simulink model "sensorsAndActuators"  (R2024a)
settings: Solver=ode2  StartTime=0.0  StopTime=inf  FixedStep=1/500  RelTol=1e-3  EnableMultiTasking=on
undefined symbols (not defined in the file): gcbh, HIL, JPEG, qc_get_step_size, video_display_show
libraries: quarc_library x32, simulink x4, simulink_extras x1
settings Model: ExtModeTrigDuration=10000  Creator=Lorena Gonzalez  LastModifiedBy=Lorena Gonzalez
settings SolverCC: AlgebraicLoopSolver=TrustRegion  PositivePriorityOrder=on
settings DataIOCC: ReturnWorkspaceOutputs=off
settings DebuggingCC: UnconnectedInputMsg=warning  UnconnectedOutputMsg=warning  UnconnectedLineMsg=warning  ArithmeticOperatorsInVariantConditions=warning
settings ModelReferenceCC: EnableRefExpFcnMdlSchedulingChecks=on
settings SFSimCC: SimUseLocalCustomCode=off  CustomCodeUndefinedFunction=UseInterfaceOnly
settings RTWCC: Description=QUARC Win64 Target Using Toolchain  SystemTargetFile=quarc_win64.tlc  TemplateMakefile=quarc_default_tmf  RTWUseLocalCustomCode=off  Toolchain=QUARC win64 | nmake (64-bit Windows)  BuildConfiguration=Faster Runs  GPUComputeCapability=3.5
settings CodeAppCC: StateflowObjectComments=on
settings STFCustomTargetCC: ConcurrentExecutionCompliant=on  SystemTargetFile=quarc_win64.tlc
settings GRTTargetCC: ParMdlRefBuildCompliant=off  CompOptLevelCompliant=off  CombineOutputUpdateFcns=off  MatFileLogging=off  CPPClassGenCompliant=off  GRTInterface=on  ExtMode=on  ExtModeMexFile=quarc_comm
settings ConfigComp: CovMetricSettings=dswe

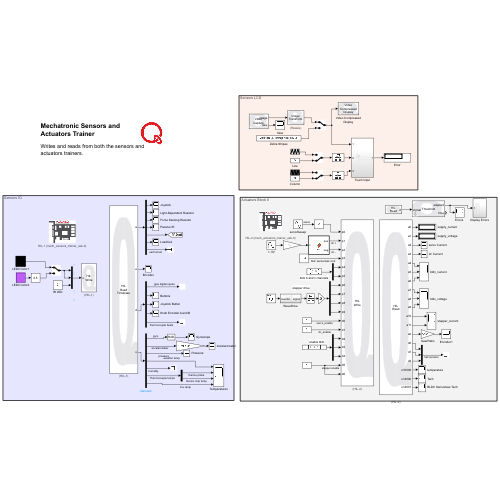
[thumbnail: Simulink's stored preview of the top-level diagram]
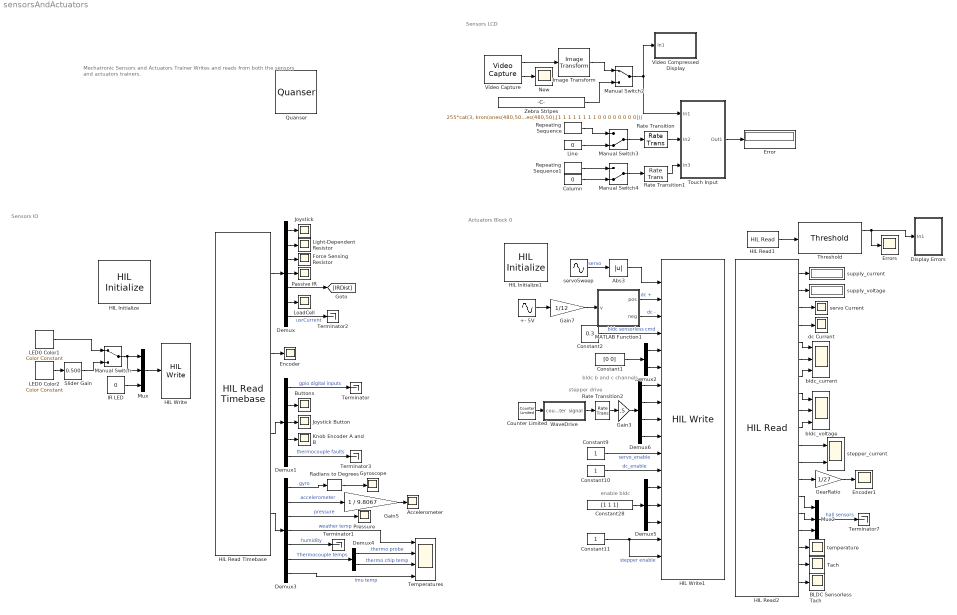
== system sensorsAndActuators ==
  note: Sensors IO
  note: Mechatronic Sensors and Actuators Trainer
      |
      | Writes and reads from both the sensors and actuators trainers.
  note: Sensors LCD
  note: enable bldc
  note: bldc b and c channels
  note: stepper drive
  note: Actuators Block 0
  +- 5V : Sin  Amplitude=5  Frequency=.75  SampleTime=0
  Abs3 : Abs  SaturateOnIntegerOverflow=off
  Accelerometer : Scope
  BLDC Sensorless Tach : Scope
  Buttons : Scope
  Column : Constant  Value=0
  Constant1 : Constant  Value=[0 0]
  Constant10 : Constant
  Constant11 : Constant
  Constant2 : Constant  Value=0.3
  Constant28 : Constant  Value=[1 1 1]
  Constant9 : Constant
  Counter Limited : simulink/Sources/Counter Limited  uplimit=3  tsamp=1/100
  Demux : Demux  Outputs=[2 1 1 1 1 1 1]
  Demux1 : Demux  Outputs=[4 2 1 2 4]
  Demux2 : Demux  Outputs=2
  Demux3 : Demux  Outputs=[3 3 1 1 2 1 1]
  Demux4 : Demux  Outputs=2
  Demux5 : Demux  Outputs=3
  Demux6 : Demux
  Display Errors : Subsystem
  Encoder : Scope
  Encoder1 : Scope
  Error : Display
  "Errors " : Scope
  Force Sensing Resistor : Scope
  Gain3 : Gain  Gain=.5
  Gain5 : Gain  Gain=1 / 9.8067
  Gain7 : Gain  Gain=1/12
  GearRatio : Gain  Gain=1/27
  Gyroscope : Scope
  HIL Initialize : quarc_library/Data Acquisition/Generic/Configuration/HIL Initialize  object_name=HIL-1  board_type=mech_sensors_trainer_usb  board_number=0  board_options=accel_avg=1;accel_filter=246;accel_fs=16;accel_rate=1125;adc1_os=64;adc2_os=64;adc3_os=16;btn0_pol=1;btn1_pol=1;color_ag=4.0;color_dg=4;color_int=50;dio0_mode=digital;dio1_mode=digital;dio2_mode=digital;dio3_mode=digital;enc_dir=0;enc_mode=encoder;enc_freq=240000000;gyro_avg=1;gyro_filter=196.6;gyro_fs=2000;gyro_rate=1125;hum_over=2;knob_dir=0;load_gain=128;load_rate=320;press_over=4;radar_bins=0;radar_down=1;radar_gain=0.3;radar_hwaas=30;radar_len=1;radar_mur=6;radar_noise=0;radar_prof=3;radar_run=0.7;radar_samp=A;radar_serv=none;radar_start=0.2;radar_sweeps=16;radar_swprate=0;temp_filter=7932;temp_over=8;tof_freq=15;tof_int=2;tof_order=close;tof_res=8x8;tof_sharp=14;ultra_int=100;ultra_len=2.4;ultra_serv=none;ultra_start=0;weather_filt=2;weather_standby=0.5;  exclusive=off  active=on  hardware_clocks=[0]  clock_modes=[]  initial_clock_frequencies=[]  set_clock_params_at_start=off  set_clock_params_at_switch_in=off  set_clock_frequencies_at_start=off  set_clock_frequencies_at_switch_in=off  analog_input_channels=[0:11]  analog_input_configurations=[]  analog_input_maximums=3.3  analog_input_minimums=0  set_analog_input_params_at_start=off  set_analog_input_params_at_switch_in=off  analog_output_channels=[]  analog_output_maximums=[]  analog_output_minimums=[]  initial_analog_outputs=[]  final_analog_outputs=[]  watchdog_analog_outputs=[]  set_analog_output_params_at_start=off  set_analog_output_params_at_switch_in=off  set_analog_outputs_at_start=off  set_analog_outputs_at_switch_in=off  set_analog_outputs_at_terminate=off  set_analog_outputs_at_switch_out=off  set_analog_outputs_on_watchdog=off  digital_input_channels=[0:30]  digital_output_channels=[]  digital_output_configuration=[]  initial_digital_outputs=[0]  final_digital_outputs=[0]  watchdog_digital_outputs=[0]  set_digital_output_params_at_start=off  set_digital_output_params_at_switch_in=off  set_digital_outputs_at_start=on  set_digital_outputs_at_switch_in=off  set_digital_outputs_at_terminate=on  set_digital_outputs_at_switch_out=off  set_digital_outputs_on_watchdog=on  encoder_channels=[0:1]  quadrature=[4]  encoder_filter_frequency=[240e6]  initial_encoder_counts=[0]  set_encoder_params_at_start=on  set_encoder_params_at_switch_in=off  set_encoder_counts_at_start=on  set_encoder_counts_at_switch_in=off  pwm_channels=[]  pwm_modes=[0]  pwm_frequency=14648.4375  pwm_configuration=[0]  pwm_alignment=[0]  pwm_polarity=[1]  pwm_leading_deadband=[]  pwm_trailing_deadband=[]  initial_pwm_outputs=[0]  final_pwm_outputs=[0]  watchdog_pwm_outputs=[0]  set_pwm_params_at_start=on  set_pwm_params_at_switch_in=off  set_pwm_outputs_at_start=on  set_pwm_outputs_at_switch_in=off  set_pwm_outputs_at_terminate=on  set_pwm_outputs_at_switch_out=off  set_pwm_outputs_on_watchdog=on  other_output_channels=[11000:11012]  initial_other_outputs=[0]  final_other_outputs=[0]  watchdog_other_outputs=[0]  set_other_outputs_at_start=on  set_other_outputs_at_switch_in=off  set_other_outputs_at_terminate=on  set_other_outputs_at_switch_out=off  set_other_outputs_on_watchdog=on
  HIL Initialize1 : quarc_library/Data Acquisition/Generic/Configuration/HIL Initialize  object_name=HIL-2  board_type=mech_actuators_trainer_usb  board_number=0  board_options=supply_voltage_low_limit=10.0;supply_voltage_high_limit=16.0;supply_current_high_limit=8.0;dc_motor_current_high_limit=1.1;servo_motor_current_high_limit=1.3;bldc_motor_current_high_limit=2.0;stepper_motor_current_high_limit=1.7;servo_pwm_range=0;enc_dir=0;bldc_motor_mode=1;bldc_start_tc=0.03;bldc_start_target=1200  exclusive=off  active=on  hardware_clocks=[0]  clock_modes=[]  initial_clock_frequencies=[]  set_clock_params_at_start=off  set_clock_params_at_switch_in=off  set_clock_frequencies_at_start=off  set_clock_frequencies_at_switch_in=off  analog_input_channels=[0:11]  analog_input_configurations=[]  analog_input_maximums=3  analog_input_minimums=-3  set_analog_input_params_at_start=off  set_analog_input_params_at_switch_in=off  analog_output_channels=[]  analog_output_maximums=[]  analog_output_minimums=[]  initial_analog_outputs=[]  final_analog_outputs=[]  watchdog_analog_outputs=[]  set_analog_output_params_at_start=off  set_analog_output_params_at_switch_in=off  set_analog_outputs_at_start=off  set_analog_outputs_at_switch_in=off  set_analog_outputs_at_terminate=off  set_analog_outputs_at_switch_out=off  set_analog_outputs_on_watchdog=off  digital_input_channels=[0:17]  digital_output_channels=[0:6]  digital_output_configuration=[]  initial_digital_outputs=[1]  final_digital_outputs=[0]  watchdog_digital_outputs=[0]  set_digital_output_params_at_start=off  set_digital_output_params_at_switch_in=off  set_digital_outputs_at_start=on  set_digital_outputs_at_switch_in=off  set_digital_outputs_at_terminate=on  set_digital_outputs_at_switch_out=off  set_digital_outputs_on_watchdog=on  encoder_channels=[0]  quadrature=[4]  encoder_filter_frequency=[]  initial_encoder_counts=[0]  set_encoder_params_at_start=on  set_encoder_params_at_switch_in=off  set_encoder_counts_at_start=on  set_encoder_counts_at_switch_in=off  pwm_channels=[0:9]  pwm_modes=[0]  pwm_frequency=23195  pwm_configuration=[1]  pwm_alignment=[0]  pwm_polarity=[1]  pwm_leading_deadband=[0]  pwm_trailing_deadband=[0]  initial_pwm_outputs=[0]  final_pwm_outputs=[0]  watchdog_pwm_outputs=[0]  set_pwm_params_at_start=off  set_pwm_params_at_switch_in=off  set_pwm_outputs_at_start=on  set_pwm_outputs_at_switch_in=off  set_pwm_outputs_at_terminate=on  set_pwm_outputs_at_switch_out=off  set_pwm_outputs_on_watchdog=on  other_output_channels=[]  initial_other_outputs=[]  final_other_outputs=[]  watchdog_other_outputs=[]  set_other_outputs_at_start=off  set_other_outputs_at_switch_in=off  set_other_outputs_at_terminate=off  set_other_outputs_at_switch_out=off  set_other_outputs_on_watchdog=off
  HIL Read Timebase : quarc_library/Data Acquisition/Generic/Timebases/HIL Read Timebase  object_name=HIL-1  clock=0  analog_channels=0:7  encoder_channels=0:1  digital_channels=[0:12]  other_channels=[3000:3002 4000:4002 9000 10000:10003 11000]  active=on  vector_output=on  data_type_mode=Inherit via back propagation  encoder_data_type=double  digital_data_type=boolean  overflow_mode=Error on overflow  samples_in_buffer=max(ceil(1/qc_get_step_size), 1)
  HIL Read1 : quarc_library/Data Acquisition/Generic/Immediate I//O/HIL Read  object_name=HIL-2  analog_channels=[]  encoder_channels=[]  digital_channels=[3:17]  other_channels=[]  sample_time=qc_get_step_size  active=on  vector_output=on  data_type_mode=Inherit via back propagation  encoder_data_type=double  digital_data_type=boolean
  HIL Read2 : quarc_library/Data Acquisition/Generic/Immediate I//O/HIL Read  object_name=HIL-2  analog_channels=[0:11]  encoder_channels=[0]  digital_channels=[0:2]  other_channels=[10000 14000:14001]  sample_time=qc_get_step_size  active=on  vector_output=off  data_type_mode=Inherit via back propagation  encoder_data_type=double  digital_data_type=boolean
  HIL Write : quarc_library/Data Acquisition/Generic/Immediate I//O/HIL Write  object_name=HIL-1  analog_channels=[]  pwm_channels=[]  digital_channels=[]  other_channels=[11000:11006]  sample_time=-1  active=off  vector_input=on
  HIL Write1 : quarc_library/Data Acquisition/Generic/Immediate I//O/HIL Write  object_name=HIL-2  analog_channels=[]  pwm_channels=[0:9]  digital_channels=[0:6]  other_channels=[]  sample_time=-1  active=off  vector_input=off
  IR LED : Constant  Value=0
  Image Transform : quarc_library/Image Processing/Generic/Image Transform  algorithm=Resize  color_theme=KRYGCBMW  min_pixel=0  max_pixel=4000  contour_depth=1  focal_length=308  principal_point=[262 334]  radial_coeffs=[-0.3129 0.0907]  tangential_coeffs=[]  extrapolated_pixel=0  interpolation=nearest  row_coords=0  column_coords=0  output_height=480  output_width=800  angle=0  origin=[240 320]  output_origin=[240 320]  output_data_type=uint8
      settings: AttributesFormatString=(%<algorithm>)  SourceProductName=QUARC Targets
  Joystick : Scope
  Joystick Button : Scope
  Knob Encoder A and B : Scope
  LED0 Color1 : quarc_library/Sources/Signals/Color Constant  color=[1 0.8 1]*0
      settings: SourceProductName=QUARC Targets
  LED0 Color2 : quarc_library/Sources/Signals/Color Constant  color=[0.75 0.36 0.98]
      settings: SourceProductName=QUARC Targets
  Light-Dependent Resistor : Scope
  Line : Constant  Value=0
  LoadCell : Scope
  MATLAB Function1 : MATLAB Function  TreatAsAtomicUnit=on
  Manual Switch : ManualSwitch
  Manual Switch2 : ManualSwitch
  Manual Switch3 : ManualSwitch  CurrentSetting=0
  Manual Switch4 : ManualSwitch  CurrentSetting=0
  Mux : Mux  Inputs=[3,3,1]
  Mux2 : Mux  Inputs=3
  New : Scope
  Passive IR : Scope
  Pressure : Scope
  Quanser : quarc_library/Logos/Quanser
  Radians to Degrees : simulink_extras/Transformations/Radians to Degrees
  Rate Transition : RateTransition  OutPortSampleTime=qc_get_step_size * ceil(1 / 30 / qc_get_step_size)
  Rate Transition1 : RateTransition  OutPortSampleTime=qc_get_step_size * ceil(1 / 30 / qc_get_step_size)
  Rate Transition2 : RateTransition
  Repeating Sequence : simulink/Sources/Repeating Sequence  rep_seq_t=[0 5 10]/5  rep_seq_y=[-200 200 -200]
  Repeating Sequence1 : simulink/Sources/Repeating Sequence  rep_seq_t=([0 5 10 15 20])/7  rep_seq_y=[-120 120 -120 120 -120]
  Slider Gain : simulink/Math Operations/Slider Gain  gain=0.500  low=0  high=1
  Tach : Scope
  Temperatures : Scope  NumInputPorts=4
  Terminator{,1..3,7} (5 alike) : Terminator
  Threshold : quarc_library/Discontinuities/Threshold  operator=>  param_src=Specify via dialog  threshold=0  duration=0.02
      settings: SourceProductName=QUARC Targets
  Touch Input : Subsystem
  Video Capture : quarc_library/Multimedia/Video Capture  source=device  device=0  filename=sample_movie.mov  value=[0 0; 0 0]  resolution=640 x 480  width=640  height=480  output_format=MATLAB RGB (HxWx3)  data_type=uint8  sample_time=qc_get_step_size * ceil(1 / 30.0 / qc_get_step_size)  brightness_override=Do not override  brightness=50.0  contrast_override=Do not override  contrast=50.0  hue_override=Do not override  hue=50.0  saturation_override=Do not override  saturation=50.0  sharpness_override=Do not override  sharpness=50.0  gamma_override=Do not override  gamma=50.0  coloreffect_override=Do not override  coloreffect=None  whitebalance_override=Do not override  whitebalance=50.0  backlightcompensation_override=Do not override  backlightcompensation=0.0  gain_override=Do not override  gain=50.0  pan_override=Do not override  pan=50.0  tilt_override=Do not override  tilt=50.0  roll_override=Do not override  roll=50.0  zoom_override=Do not override  zoom=0.0  exposure_override=Do not override  exposure=50.0  iris_override=Do not override  iris=50.0  mirror_override=Do not override  mirror=None  focus_override=Do not override  focus=0.0
      settings: SourceProductName=QUARC Targets
  Video Compressed Display : Subsystem  LoadFcn=set_param(gcbh, 'UserData', gcb);  StartFcn=video_display_show([gcb, '/Video Display'], 'add', gcb);  mask(Video Compressed Display){algorithm=JPEG, quality=50, sample_time=-1, use_hardware=on}
      mask prompts: algorithm "Compression algorithm:"; quality "Compression quality (0-100):"; sample_time "Sample time (seconds):"; use_hardware "Use hardware acceleration for video display"
      mask help: Displays a video stream on the host, using compression to minimize bandwidth.
      mask init:
      | qc_set_display('Video\nCompressed\nDisplay');
      settings: UndoDeleteFcn=set_param(gcbh, 'UserData', gcb);  OpenFcn=video_display_show([gcb, '/Video Display'], 'show', gcb);  PreDeleteFcn=video_display_show([gcb, '/Video Display'], 'delete');
      settings: CopyFcn=|
      | set_param(gcbh, 'UserData', gcb);
      | set_param(gcbh, 'LinkStatus', 'none');
      settings: NameChangeFcn=|
      | video_display_show([get_param(gcbh, 'UserData'), '/Video Display'], 'rename', [gcb, '/Video Display']);
      | video_display_show([gcb, '/Video Display'], 'add', gcb);
      | set_param(gcbh, 'UserData', gcb);
      mask Help: web(qc_get_block_help_path(gcb));
      mask TypeOptions algorithm: Image Compress/algorithm
      mask TypeOptions quality: Image Compress/quality
      mask TypeOptions sample_time: Video Display/sample_time
      mask TypeOptions use_hardware: Video Display/use_hardware
      mask Display:
      | patch([0.98591 0.98591 0.62618 0.59072 0.56147   0.536   0.536  0.5441 0.56912 0.59207 0.60881 0.62276 0.63527 0.64364  0.6485  0.6485 0.64706 0.64499 0.63662 0.62411 0.61232 0.59837 0.58307 0.56147   0.536   0.536  0.5441  0.5747 0.60953 0.63662 0.67001  0.7034 0.72851 0.75425 0.77927 0.80294 0.82454 0.84119 0.85865 0.87395 0.88574 0.89339  0.8969 0.89969 0.89969 0.89267  0.8816 0.87044 0.85649  0.8384 0.81824 0.80294 0.78764 0.77513 0.76676 0.75776 0.76397 0.77513 0.79178 0.80987 0.82796 0.84326 0.86207 0.98528],[0.18689 0.05522 0.05522 0.05171 0.05171    0.05 0.18338 0.18338 0.19148 0.20435 0.22298 0.24863 0.28589 0.33125 0.38138 0.55139 0.59801 0.63761 0.68189 0.72149 0.74939 0.76694 0.77855 0.79367 0.79952 0.92768 0.92768 0.92768 0.92417 0.92066 0.91364  0.9032 0.89384 0.88106 0.86594 0.85073 0.82634 0.80537 0.77855 0.74363 0.70403 0.65858 0.61079 0.59099 0.41513 0.37202 0.31847 0.29048 0.25556 0.23342  0.2102 0.19382 0.18221 0.17285 0.16943 0.16124  0.1589 0.16241 0.16709 0.17168  0.1787 0.18221 0.18689 0.18689],[0.9,0.90,0.91])
      | patch([0.536 0.52601 0.46823 0.44528 0.41603 0.39101 0.35555 0.33116 0.31451 0.29291  0.2804 0.26717 0.25322 0.23999 0.22406 0.20732 0.19337 0.17528 0.15935 0.14396 0.13217 0.11759 0.10922 0.10085 0.09671 0.09392 0.09041 0.08906 0.08906 0.09464  0.0995 0.10778 0.11894 0.13145 0.14675 0.16349 0.17672 0.19409 0.20732 0.22406 0.23999 0.26159 0.27833 0.29849 0.31793 0.33602 0.35411 0.37085 0.39245 0.41603   0.536   0.536 0.53159 0.46409   0.446 0.42026 0.39587 0.37571 0.36113 0.34925 0.34088 0.33809 0.33809 0.34088 0.34583 0.35627 0.36392 0.38129 0.39587 0.41117 0.42719 0.44672  0.4676 0.48353 0.48353 0.52394   0.536],[0.05 0.04829 0.04712 0.04712 0.04829 0.05063 0.05405 0.05873 0.06107 0.06692 0.07043 0.07619 0.08087 0.08672 0.09482 0.10652 0.11696 0.13325  0.1508 0.17168 0.19499 0.22415 0.25439 0.28472 0.31379 0.35456 0.38489 0.41513 0.58055 0.63878 0.68774 0.72149 0.75641 0.78089 0.80537 0.82859 0.84029 0.85658 0.86594 0.87404  0.8834 0.89267 0.90086 0.90788 0.91247 0.91832 0.92066   0.923 0.92651 0.92768 0.92768 0.79952 0.79952 0.79952 0.79718 0.78899 0.77153 0.75056 0.72149 0.68072 0.62249  0.5549 0.41396 0.37085 0.33242 0.28121 0.25205 0.22181 0.20552 0.19499 0.18572 0.18221 0.17753 0.17636 0.17753  0.1787  0.1787],[0.9,0.90,0.91])
      | disp('Video\nCompressed\nDisplay');
  WaveDrive : Subsystem
  Zebra Stripes : Constant  Value=255*cat(3, kron(ones(480,50),[1 1 1 1 1 1 1 1 0 0 0 0 0 0 0 0]),kron(ones(480,50),[1 1 1 1 1 1 1 1 0 0 0 0 0 0 0 0]),kron(ones(480,50),[1 1 1 1 1 1 1 1 0 0 0 0 0 0 0 0]))  OutDataTypeStr=uint8
  bldc_current : Scope  NumInputPorts=3
  bldc_voltage : Scope  NumInputPorts=3
  dc Current : Scope
  servo Current : Scope
  servoSweep : Sin  SampleTime=0
  stepper_current : Scope  NumInputPorts=2
  supply_current : Display
  supply_voltage : Display
  temperature : Scope
  wires:
  Rate Transition1/1 -> Touch Input/3(In3)
  Video Capture/1 -> Image Transform/1
  Demux3/2 -> Gain5/1  "accelerometer"
  Image Transform/1 -> Manual Switch2/1
  Radians to Degrees/1 -> Gyroscope/1
  Manual Switch3/1 -> Rate Transition/1
  Demux/7 -> Terminator2/1  "usrCurrent"
  Demux1/5 -> Terminator3/1  "thermocouple faults"
  Repeating Sequence1/1 -> Manual Switch4/1
  Repeating Sequence/1 -> Manual Switch3/1
  Demux4/1 -> Temperatures/2  "thermo probe"
  Demux1/4 -> Knob Encoder A and B/1
  Touch Input/1(Out1) -> Error/1
  Rate Transition/1 -> Touch Input/2(In2)
  HIL Read Timebase/1 -> Demux/1
  Slider Gain/1 -> Manual Switch/2
  Demux/6 -> LoadCell/1
  Demux1/1 -> Terminator/1  "gpio digital inputs"
  Demux/3 -> Force Sensing Resistor/1
  Demux3/1 -> Radians to Degrees/1  "gyro"
  LED0 Color2/1 -> Slider Gain/1
  LED0 Color1/1 -> Manual Switch/1
  Manual Switch/1 -> Mux/2, Mux/1
  Demux/2 -> Light-Dependent Resistor/1
  Demux3/6 -> Demux4/1  "Thermocouple temps"
  Demux4/2 -> Temperatures/3  "thermo chip temp"
  IR LED/1 -> Mux/3
  Gain5/1 -> Accelerometer/1
  Demux1/3 -> Joystick Button/1
  Video Capture/2 -> New/1
  Demux/5 -> [IRDist]
  Demux/1 -> Joystick/1
  Line/1 -> Manual Switch3/2
  Manual Switch4/1 -> Rate Transition1/1
  Demux3/3 -> Pressure/1  "pressure"
  Mux/1 -> HIL Write/1
  Demux/4 -> Passive IR/1
  Demux3/4 -> Temperatures/1  "weather temp"
  Demux3/7 -> Temperatures/4  "imu temp"
  HIL Read Timebase/2 -> Encoder/1
  Manual Switch2/1 -> Touch Input/1(In1), Video Compressed Display/1(In1)
  HIL Read Timebase/3 -> Demux1/1
  Zebra Stripes/1 -> Manual Switch2/2
  Column/1 -> Manual Switch4/2
  HIL Read Timebase/4 -> Demux3/1
  Demux1/2 -> Buttons/1
  HIL Read2/18 -> Tach/1
  Abs3/1 -> HIL Write1/1
  HIL Read2/4 -> dc Current/1
  HIL Read2/19 -> BLDC Sensorless Tach/1
  Demux5/1 -> HIL Write1/13
  Demux5/2 -> HIL Write1/14
  Threshold/1 -> Display Errors/1(In1), "Errors "/1
  GearRatio/1 -> Encoder1/1
  Constant11/1 -> HIL Write1/16, HIL Write1/17  "stepper enable"
  Constant9/1 -> HIL Write1/11  "servo_enable"
  MATLAB Function1/2(neg) -> HIL Write1/3  "dc -"
  MATLAB Function1/1(pos) -> HIL Write1/2  "dc +"
  Demux6/2 -> HIL Write1/8
  Demux2/2 -> HIL Write1/6
  HIL Read2/12 -> stepper_current/2
  Demux2/1 -> HIL Write1/5
  HIL Read2/13 -> GearRatio/1
  Gain7/1 -> MATLAB Function1/1(v)
  Gain3/1 -> Demux6/1
  servoSweep/1 -> Abs3/1  "servo"
  +- 5V/1 -> Gain7/1
  WaveDrive/1(signal) -> Rate Transition2/1
  Demux6/3 -> HIL Write1/9
  Mux2/1 -> Terminator7/1  "hall sensors"
  HIL Read2/10 -> bldc_voltage/3
  HIL Read2/17 -> temperature/1
  HIL Read2/8 -> bldc_voltage/1
  HIL Read2/9 -> bldc_voltage/2
  Constant28/1 -> Demux5/1
  Demux5/3 -> HIL Write1/15
  HIL Read2/16 -> Mux2/3
  Counter Limited/1 -> WaveDrive/1(counter)
  Constant2/1 -> HIL Write1/4  "bldc sensorless cmd"
  HIL Read2/15 -> Mux2/2
  HIL Read2/2 -> supply_voltage/1
  HIL Read2/5 -> bldc_current/1
  HIL Read2/11 -> stepper_current/1
  HIL Read2/7 -> bldc_current/3
  Constant1/1 -> Demux2/1
  Constant10/1 -> HIL Write1/12  "dc_enable"
  Rate Transition2/1 -> Gain3/1
  Demux6/4 -> HIL Write1/10
  HIL Read2/1 -> supply_current/1
  HIL Read1/1 -> Threshold/1
  HIL Read2/14 -> Mux2/1
  HIL Read2/6 -> bldc_current/2
  Demux6/1 -> HIL Write1/7
  HIL Read2/3 -> servo Current/1
  Demux3/5 -> Terminator1/1  "humidity"

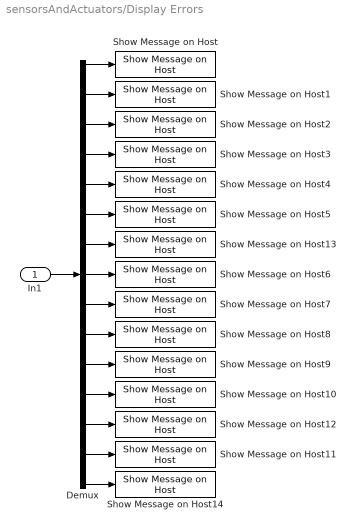
== system sensorsAndActuators/Display Errors ==
  In1 : Inport
  Demux : Demux  Outputs=15
  Show Message on Host : quarc_library/Sinks/Error Handling/Show Message on Host  message_type=Fixed error message  message_icon=Error  message=Power Supply Voltage Too Low
      settings: AttributesFormatString="\"%<message>\""  SourceProductName=QUARC Targets
  Show Message on Host1 : quarc_library/Sinks/Error Handling/Show Message on Host  message_type=Fixed error message  message_icon=Error  message=Power Supply Voltage Too High
      settings: AttributesFormatString="\"%<message>\""  SourceProductName=QUARC Targets
  Show Message on Host10 : quarc_library/Sinks/Error Handling/Show Message on Host  message_type=Fixed error message  message_icon=Error  message=Stepper Channel B Current Too High
      settings: AttributesFormatString="\"%<message>\""  SourceProductName=QUARC Targets
  Show Message on Host11 : quarc_library/Sinks/Error Handling/Show Message on Host  message_type=Fixed error message  message_icon=Error  message=Stepper Channel B Driver Over Current/Temperature
      settings: AttributesFormatString="\"%<message>\""  SourceProductName=QUARC Targets
  Show Message on Host12 : quarc_library/Sinks/Error Handling/Show Message on Host  message_type=Fixed error message  message_icon=Error  message=Stepper Channel A Driver Over Current/Temperature
      settings: AttributesFormatString="\"%<message>\""  SourceProductName=QUARC Targets
  Show Message on Host13 : quarc_library/Sinks/Error Handling/Show Message on Host  message_type=Fixed error message  message_icon=Error  message=Servo Motor Voltage Out of Range
      settings: AttributesFormatString="\"%<message>\""  SourceProductName=QUARC Targets
  Show Message on Host14 : quarc_library/Sinks/Error Handling/Show Message on Host  message_type=Fixed error message  message_icon=Error  message=Device Over-Temperature
      settings: AttributesFormatString="\"%<message>\""  SourceProductName=QUARC Targets
  Show Message on Host2 : quarc_library/Sinks/Error Handling/Show Message on Host  message_type=Fixed error message  message_icon=Error  message=Power Supply Current Too High
      settings: AttributesFormatString="\"%<message>\""  SourceProductName=QUARC Targets
  Show Message on Host3 : quarc_library/Sinks/Error Handling/Show Message on Host  message_type=Fixed error message  message_icon=Error  message=DC Motor Current Too High
      settings: AttributesFormatString="\"%<message>\""  SourceProductName=QUARC Targets
  Show Message on Host4 : quarc_library/Sinks/Error Handling/Show Message on Host  message_type=Fixed error message  message_icon=Error  message=DC Motor Driver Over Current/Temperature
      settings: AttributesFormatString="\"%<message>\""  SourceProductName=QUARC Targets
  Show Message on Host5 : quarc_library/Sinks/Error Handling/Show Message on Host  message_type=Fixed error message  message_icon=Error  message=Servo Motor Current Too High
      settings: AttributesFormatString="\"%<message>\""  SourceProductName=QUARC Targets
  Show Message on Host6 : quarc_library/Sinks/Error Handling/Show Message on Host  message_type=Fixed error message  message_icon=Error  message=BLDC Channel A Current Too High
      settings: AttributesFormatString="\"%<message>\""  SourceProductName=QUARC Targets
  Show Message on Host7 : quarc_library/Sinks/Error Handling/Show Message on Host  message_type=Fixed error message  message_icon=Error  message=BLDC Channel B Current Too High
      settings: AttributesFormatString="\"%<message>\""  SourceProductName=QUARC Targets
  Show Message on Host8 : quarc_library/Sinks/Error Handling/Show Message on Host  message_type=Fixed error message  message_icon=Error  message=BLDC Channel C Current Too High
      settings: AttributesFormatString="\"%<message>\""  SourceProductName=QUARC Targets
  Show Message on Host9 : quarc_library/Sinks/Error Handling/Show Message on Host  message_type=Fixed error message  message_icon=Error  message=Stepper Channel A Current Too High
      settings: AttributesFormatString="\"%<message>\""  SourceProductName=QUARC Targets
  wires:
  In1/1 -> Demux/1
  Demux/1 -> Show Message on Host/1
  Demux/2 -> Show Message on Host1/1
  Demux/3 -> Show Message on Host2/1
  Demux/4 -> Show Message on Host3/1
  Demux/5 -> Show Message on Host4/1
  Demux/6 -> Show Message on Host5/1
  Demux/8 -> Show Message on Host6/1
  Demux/9 -> Show Message on Host7/1
  Demux/10 -> Show Message on Host8/1
  Demux/11 -> Show Message on Host9/1
  Demux/12 -> Show Message on Host10/1
  Demux/13 -> Show Message on Host12/1
  Demux/14 -> Show Message on Host11/1
  Demux/15 -> Show Message on Host14/1
  Demux/7 -> Show Message on Host13/1

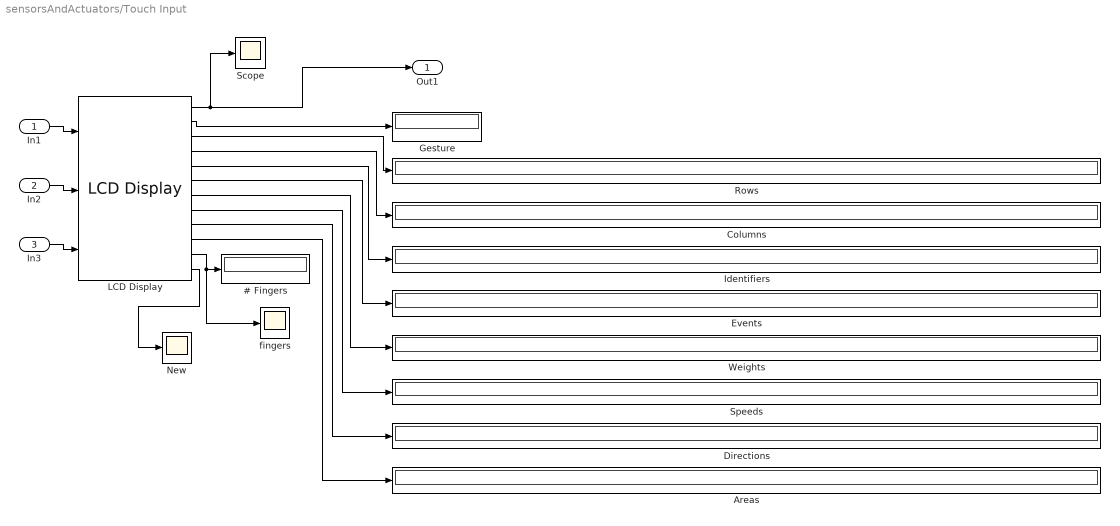
== system sensorsAndActuators/Touch Input ==
  In1 : Inport
  In2 : Inport  Port=2
  In3 : Inport  Port=3
  # Fingers : Display
  Areas : Display
  Columns : Display
  Directions : Display
  Events : Display
  Gesture : Display
  Identifiers : Display
  LCD Display : quarc_library/Devices/Third-Party/Displays/LCD Display  display_type=Quanser Mechatronics Sensors Trainer USB LCD  mode=image  uri=lcd://localhost:0  sample_time=-1  output_sample_time=qc_get_step_size * ceil(1 / 60 / qc_get_step_size)  dark_mode=on  rotate=off  active=on
      settings: SourceProductName=QUARC Targets
  New : Scope
  Rows : Display
  Scope : Scope
  Speeds : Display
  Weights : Display
  fingers : Scope
  Out1 : Outport
  wires:
  LCD Display/1 -> Scope/1, Out1/1
  In3/1 -> LCD Display/3
  In2/1 -> LCD Display/2
  In1/1 -> LCD Display/1
  LCD Display/2 -> Gesture/1
  LCD Display/3 -> Rows/1
  LCD Display/4 -> Columns/1
  LCD Display/5 -> Identifiers/1
  LCD Display/6 -> Events/1
  LCD Display/7 -> Weights/1
  LCD Display/8 -> Speeds/1
  LCD Display/9 -> Directions/1
  LCD Display/10 -> Areas/1
  LCD Display/11 -> fingers/1, # Fingers/1
  LCD Display/12 -> New/1

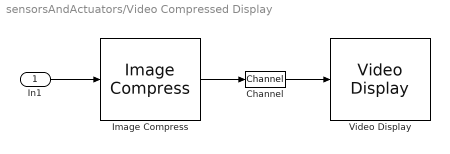
== system sensorsAndActuators/Video Compressed Display ==
  In1 : Inport
  Channel : quarc_library/Signal Routing/Channel  channel=1  buffer_size=1
  Image Compress : quarc_library/Image Processing/Generic/Image Compress  algorithm=JPEG  source=Internal dialog parameter  quality=quality  output_dim=-1
  Video Display : quarc_library/Multimedia/Video Display  Tag=sensorsAndActuators/Video Compressed Display/Video Display  sample_time=sample_time  use_hardware=on
  wires:
  Image Compress/1 -> Channel/1
  In1/1 -> Image Compress/1
  Channel/1 -> Video Display/1

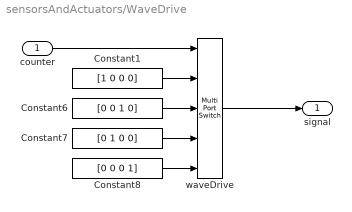
== system sensorsAndActuators/WaveDrive ==
  counter : Inport
  Constant1 : Constant  Value=[1 0 0 0]
  Constant6 : Constant  Value=[0 0 1 0]
  Constant7 : Constant  Value=[0 1 0 0]
  Constant8 : Constant  Value=[0 0 0 1]
  waveDrive : MultiPortSwitch  Inputs=4  SaturateOnIntegerOverflow=off  InputSameDT=off
  signal : Outport
  wires:
  Constant6/1 -> waveDrive/3
  Constant7/1 -> waveDrive/4
  counter/1 -> waveDrive/1
  waveDrive/1 -> signal/1
  Constant8/1 -> waveDrive/5
  Constant1/1 -> waveDrive/2

== matlab function sensorsAndActuators/MATLAB Function1 ==
  data: v input; pos output; neg output
function [pos, neg]= fcn(v)

if v >= 0
    pos = v;
    neg = 0;
else
    pos = 0;
    neg = abs(v);
end
